simulink subsystem "PvtSubSys_PLAN_ALL"  (R2020b)
settings: Solver=VariableStepAuto  StartTime=0.0  StopTime=10.0  RelTol=1e-3
libraries: simulink x1
settings Model: Creator=Cheng  LastModifiedBy=Cheng

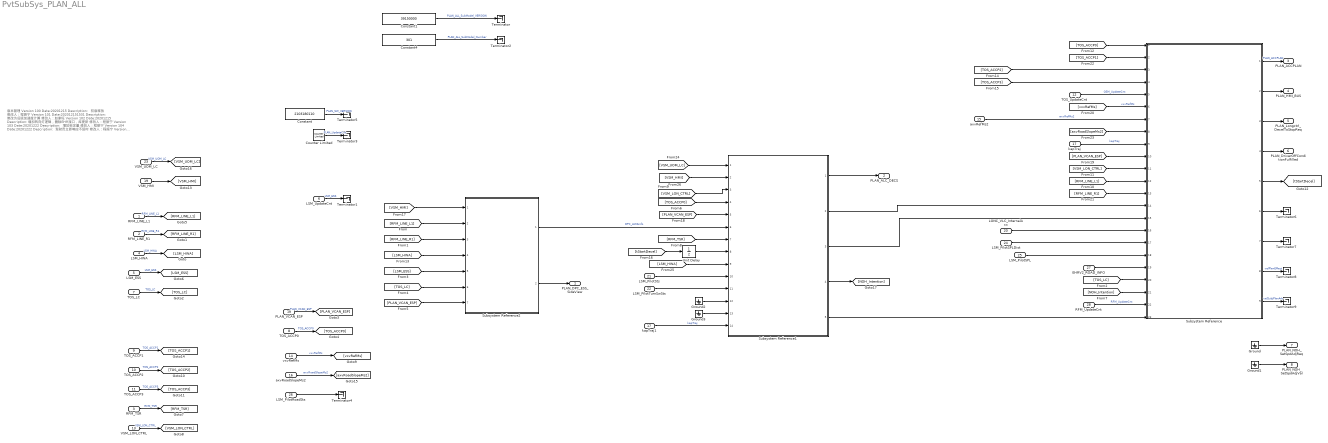
== system PvtSubSys_PLAN_ALL ==
  note: 版本管理
      | Version 100
      | Date:20201215
      | Description: 初版释放
      | 修改人：程振宁
      |
      | Version 101
      | Date:202012151531
      | Description: 修改为旧版加速度计算
      | 修改人：赵家旺
      |
      | Version 102
      | Date:20201215
      | Description: 增加转向灯逻辑，删除EHR接口，库更新
      | 修改人：程振宁
      |
      | Version 103
      | Date:20201222
      | Description: 增加标定量
      | 修改人：程振宁
      |
      | Version 104
      | Date:20201222
      | Description: 驾驶员立即响应不延时
      | 修改人：程振宁
      |
      | Version 105
      | Date:20201229
      | Description: 拆分
      | 修改人：程振宁
      |
      | Version 106
      | Date:20210106
      | Description: 接口修改
      | 修改人：程振宁
      |
      | Version 2103150109
      | Date:20210315
      | Description: PLAN添加EHRV2接口
      | 修改人：赵家旺
      |
      | Version 2103180110
      | Date:20210318
      | Description: PLAN添加RFM_UpdateCnt接口
      | 修改人：赵家旺
  RFM_LINE_L1 : Inport  OutDataTypeStr=Bus: RFM_LINE_BUS  PortDimensions=1  Interpolate=off  BusOutputAsStruct=on
  RFM_LINE_R1 : Inport  Port=2  OutDataTypeStr=Bus: RFM_LINE_BUS  PortDimensions=1  Interpolate=off  BusOutputAsStruct=on
  RFM_TSR : Inport  Port=3  OutDataTypeStr=Bus: RFM_TSR_BUS  PortDimensions=1  Interpolate=off  BusOutputAsStruct=on
  LSM_HWA : Inport  Port=4  OutDataTypeStr=Bus: LSM_HWA_BUS  PortDimensions=1  Interpolate=off  BusOutputAsStruct=on
  LSM_ESS : Inport  Port=5  OutDataTypeStr=Bus: LSM_ESS_BUS  PortDimensions=1  Interpolate=off  BusOutputAsStruct=on
  LSM_UpdateCnt : Inport  Port=6  OutDataTypeStr=uint32  PortDimensions=1  Interpolate=off  BusOutputAsStruct=on
  TOS_LC : Inport  Port=7  OutDataTypeStr=Bus: TOS_LC_BUS  PortDimensions=1  BusOutputAsStruct=on
  TOS_ACCP0 : Inport  Port=8  OutDataTypeStr=Bus: TOS_ACCP0_BUS  PortDimensions=1  BusOutputAsStruct=on
  TOS_ACCP1 : Inport  Port=9  OutDataTypeStr=Bus: TOS_ACCP1_BUS  LockScale=on
  TOS_ACCP2 : Inport  Port=10  OutDataTypeStr=Bus: TOS_ACCP2_BUS
  TOS_ACCP3 : Inport  Port=11  OutDataTypeStr=Bus: TOS_ACCP3_BUS
  TOS_UpdateCnt : Inport  Port=12
  VSM_LON_CTRL : Inport  Port=13  OutDataTypeStr=Bus: VSM_LON_CTRL_BUS  PortDimensions=1  Interpolate=off  BusOutputAsStruct=on
  vxvRefMs : Inport  Port=14  OutDataTypeStr=single  PortDimensions=1  Interpolate=off  BusOutputAsStruct=on
  axvRefMs2 : Inport  Port=15
  axvRoadSlopeMs2 : Inport  Port=16
  kapTraj : Inport  Port=17
  PLAN_VCAN_ESP : Inport  Port=18  OutDataTypeStr=Bus: VCAN_ESP_MSG_BUS
  VSM_HMI : Inport  Port=19  OutDataTypeStr=Bus: VSM_HMI_BUS
  LONC_VLC_InternalAcc : Inport  Port=20  OutDataTypeStr=single
  LSM_PilotSts : Inport  Port=21
  LSM_PilotTurnSwSts : Inport  Port=22
  VSM_UOM_LC : Inport  Port=23  OutDataTypeStr=Bus: VSM_UOM_LC_BUS
  LSM_PilotSPLDist : Inport  Port=24  OutDataTypeStr=uint16
  LSM_PilotSPL : Inport  Port=25  OutDataTypeStr=uint8
  LSM_PilotRoadSts : Inport  Port=26  OutDataTypeStr=uint8
  EHRV2_ROAD_INFO : Inport  Port=27  OutDataTypeStr=Bus: EHRV2_ROAD_INFO_BUS
  RFM_UpdateCnt : Inport  Port=28
  Constant : Constant  Value=2103180110  OutDataTypeStr=uint32
  Constant1 : Constant  Value=39150000  OutDataTypeStr=uint32
  Constant4 : Constant  Value=301  OutDataTypeStr=uint32
  Counter Limited : simulink/Sources/Counter Limited  uplimit=255  tsamp=-1
  Ground{,1..3} (4 alike) : Ground
  Subsystem Reference : Subsystem  ReferencedSubsystem=PvtSubSys_PLAN_AP
  Subsystem Reference1 : Subsystem  ReferencedSubsystem=PvtSubSys_PLAN_ALC
  Subsystem Reference2 : Subsystem  ReferencedSubsystem=PvtSubSys_PLAN_DPC
  Terminator{,1..9} (10 alike) : Terminator
  Unit Delay : UnitDelay  SampleTime=-1  HasFrameUpgradeWarning=on
  kapTraj1 : InportShadow  Port=17
  PLAN_DPC_ESS_SideView : Outport  OutDataTypeStr=Bus: PLAN_DPC_ESS_BUS
  PLAN_ALC_DECS : Outport  Port=2  OutDataTypeStr=Bus: PLAN_ALC_DECS_BUS
  PLAN_ACCPLAN : Outport  Port=3  OutDataTypeStr=Bus: PLAN_ACCPLAN_BUS
  PLAN_HMI_BUS : Outport  Port=4  OutDataTypeStr=Bus: PLAN_HMI_BUS
  PLAN_Longctrl_DecelToStopReq : Outport  Port=5  OutDataTypeStr=boolean
  PLAN_DriverOffConditionFulfilled : Outport  Port=6  OutDataTypeStr=boolean
  PLAN_NOH_SetSpdAdjReq : Outport  Port=7  OutDataTypeStr=boolean
  PLAN_NOH_SetSpdAdjVal : Outport  Port=8  OutDataTypeStr=uint8
  wires:
  Constant1/1 -> Terminator/1  "PLAN_ALL_SubModel_VERSION"
  Constant4/1 -> Terminator2/1  "PLAN_ALL_SubModel_Number"
  [vxvRefMs] -> Subsystem Reference/6  "vxvRefMs"
  PLAN_VCAN_ESP/1 -> [PLAN_VCAN_ESP]  "PLAN_VCAN_ESP"
  Constant/1 -> Terminator5/1  "PLAN_SW_VERSION"
  TOS_LC/1 -> [TOS_LC]  "TOS_LC"
  TOS_UpdateCnt/1 -> Subsystem Reference/5  "OSM_UpdateCnt"
  [tStartDecel] -> Unit Delay/1
  RFM_LINE_R1/1 -> [RFM_LINE_R1]  "RFM_LINE_R1"
  VSM_HMI/1 -> [VSM_HMI]
  LSM_UpdateCnt/1 -> Terminator1/1  "LSM_ESS"
  TOS_ACCP0/1 -> [TOS_ACCP0]  "TOS_ACCP0"
  vxvRefMs/1 -> [vxvRefMs]  "vxvRefMs"
  axvRoadSlopeMs2/1 -> [axvRoadSlopeMs2]  "axvRoadSlopeMs2"
  RFM_LINE_L1/1 -> [RFM_LINE_L1]  "RFM_LINE_L1"
  VSM_UOM_LC/1 -> [VSM_UOM_LC]  "VSM_UOM_LC"
  [PLAN_VCAN_ESP] -> Subsystem Reference/10
  kapTraj/1 -> Subsystem Reference/9  "kapTraj"
  LSM_PilotRoadSts/1 -> Terminator4/1
  Subsystem Reference/4 -> PLAN_DriverOffConditionFulfilled/1
  LONC_VLC_InternalAcc/1 -> Subsystem Reference/16
  kapTraj1/1 -> Subsystem Reference1/14  "kapTraj"
  TOS_ACCP3/1 -> [TOS_ACCP3]  "TOS_ACCP3"
  RFM_UpdateCnt/1 -> Subsystem Reference/22  "RFM_UpdateCnt"
  [TOS_ACCP2] -> Subsystem Reference/3
  Subsystem Reference1/5 -> Subsystem Reference/23
  Subsystem Reference1/1 -> PLAN_ALC_DECS/1
  [VSM_LON_CTRL] -> Subsystem Reference/11
  Subsystem Reference1/4 -> [NOH_Intention]
  Counter Limited/1 -> Terminator3/1  "PLAN_UpdateCnt"
  [TOS_LC] -> Subsystem Reference/20
  EHRV2_ROAD_INFO/1 -> Subsystem Reference/19
  Ground/1 -> PLAN_NOH_SetSpdAdjReq/1
  LSM_PilotSPL/1 -> Subsystem Reference/18
  Subsystem Reference/1 -> PLAN_ACCPLAN/1  "PLAN_ACCPLAN"
  Subsystem Reference1/3 -> Subsystem Reference/15
  [TOS_ACCP3] -> Subsystem Reference/4
  Subsystem Reference1/2 -> Subsystem Reference/14
  axvRefMs2/1 -> Subsystem Reference/7  "axvRefMs2"
  [TOS_ACCP0] -> Subsystem Reference/1
  LSM_ESS/1 -> [LSM_ESS]  "LSM_ESS"
  [RFM_LINE_R1] -> Subsystem Reference/13
  TOS_ACCP2/1 -> [TOS_ACCP2]  "TOS_ACCP2"
  Subsystem Reference/2 -> PLAN_HMI_BUS/1
  Subsystem Reference/6 -> Terminator6/1
  RFM_TSR/1 -> [RFM_TSR]  "RFM_TSR"
  Subsystem Reference/7 -> Terminator7/1
  LSM_HWA/1 -> [LSM_HWA]  "LSM_HWA"
  Subsystem Reference2/2 -> PLAN_DPC_ESS_SideView/1
  [NOH_Intention] -> Subsystem Reference/21
  Subsystem Reference/3 -> PLAN_Longctrl_DecelToStopReq/1
  TOS_ACCP1/1 -> [TOS_ACCP1]  "TOS_ACCP1"
  Ground1/1 -> PLAN_NOH_SetSpdAdjVal/1
  LSM_PilotSPLDist/1 -> Subsystem Reference/17
  VSM_LON_CTRL/1 -> [VSM_LON_CTRL]  "VSM_LON_CTRL"
  [TOS_ACCP1] -> Subsystem Reference/2
  [axvRoadSlopeMs2] -> Subsystem Reference/8
  Subsystem Reference/5 -> [tStartDecel]
  [RFM_LINE_L1] -> Subsystem Reference/12
  [LSM_HWA] -> Subsystem Reference2/4
  [VSM_HMI] -> Subsystem Reference2/1
  Ground2/1 -> Subsystem Reference1/12
  Subsystem Reference2/1 -> Subsystem Reference1/6  "DPC_HWAinfo"
  [VSM_LON_CTRL] -> Subsystem Reference1/3
  Unit Delay/1 -> Subsystem Reference1/8
  [RFM_TSR] -> Subsystem Reference1/7
  LSM_PilotSts/1 -> Subsystem Reference1/10
  [VSM_UOM_LC] -> Subsystem Reference1/1
  [RFM_LINE_R1] -> Subsystem Reference2/3
  [TOS_LC] -> Subsystem Reference2/6
  [LSM_ESS] -> Subsystem Reference2/5
  Ground3/1 -> Subsystem Reference1/13
  LSM_PilotTurnSwSts/1 -> Subsystem Reference1/11
  [TOS_ACCP0] -> Subsystem Reference1/4
  [RFM_LINE_L1] -> Subsystem Reference2/2
  [PLAN_VCAN_ESP] -> Subsystem Reference2/7
  [PLAN_VCAN_ESP] -> Subsystem Reference1/5
  [LSM_HWA] -> Subsystem Reference1/9
  [VSM_HMI] -> Subsystem Reference1/2
  Subsystem Reference/8 -> Terminator8/1  "velPlanEffect"
  Subsystem Reference/9 -> Terminator9/1  "velSubjPlanArb"
